simulink model "RVC_Joint_space_PD_control_gravity_compensation"  (R2020b)
settings: Solver=VariableStepAuto  StartTime=0.0  StopTime=5  RelTol=1e-3
values from neighbouring files (symbols this model uses):
  gravity = [0 0 9.81]'    [RVC_main.m]
  KD_J = diag([1 1 1 0.1 0.1 0.1])    [RVC_main.m]
  KP_J = diag([0.5 0.5 0.5 0.25 0.255 0.25])    [RVC_main.m]
undefined symbols (not defined in the file or in its folder): dh, inv_dyn_recursive_NewtonEulero
libraries: vrlib x1
settings Model: Creator=eros  LastModifiedBy=Edoardo

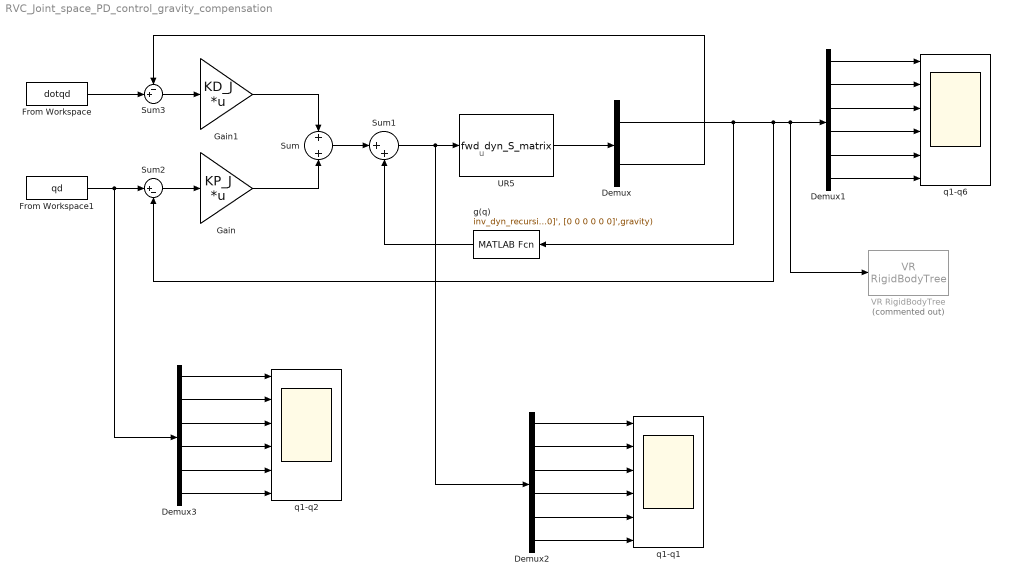
== system RVC_Joint_space_PD_control_gravity_compensation ==
  note: u
  Demux : Demux  Outputs=2
  Demux1 : Demux  Outputs=dh.dof
  Demux2 : Demux  Outputs=dh.dof
  Demux3 : Demux  Outputs=dh.dof
  From Workspace : FromWorkspace  VariableName=dotqd
  From Workspace1 : FromWorkspace  VariableName=qd
  Gain : Gain  Gain=KP_J  Multiplication=Matrix(K*u)
  Gain1 : Gain  Gain=KD_J  Multiplication=Matrix(K*u)
  Sum : Sum
  Sum1 : Sum  Inputs=|++
  Sum2 : Sum  Inputs=|+-
  Sum3 : Sum  Inputs=-+|
  UR5 : S-Function  FunctionName=fwd_dyn_S_matrix  Parameters=dh, he, gravity, q0, dotq0  SFunctionDeploymentMode=off  EnableBusSupport=off
  VR RigidBodyTree : vrlib/VR RigidBodyTree  Commented=on  RBT=UR5_robot  useRBT=on  Ts=-1  ForceViewerOpen=on
      settings: SourceProductBaseCode=SL
  g(q) : MATLABFcn  MATLABFcn=inv_dyn_recursive_NewtonEulero(dh,u,[0 0 0 0 0 0]', [0 0 0 0 0 0]',gravity)  OutputDimensions=[dh.dof 1]  Output1D=off
  q1-q1 : Scope  NumInputPorts=6
  q1-q2 : Scope  NumInputPorts=6
  q1-q6 : Scope  NumInputPorts=6
  wires:
  Sum/1 -> Sum1/1
  g(q)/1 -> Sum1/2
  Gain/1 -> Sum/2
  UR5/1 -> Demux/1
  Demux/1 -> Sum2/2, VR RigidBodyTree/1, Demux1/1, g(q)/1
  Sum2/1 -> Gain/1
  Gain1/1 -> Sum/1
  Demux1/1 -> q1-q6/1
  Demux1/2 -> q1-q6/2
  Demux1/3 -> q1-q6/3
  Demux1/4 -> q1-q6/4
  Demux1/5 -> q1-q6/5
  Demux1/6 -> q1-q6/6
  From Workspace/1 -> Sum3/2
  Demux/2 -> Sum3/1
  Sum3/1 -> Gain1/1
  Demux2/3 -> q1-q1/3
  Demux2/1 -> q1-q1/1
  Demux2/5 -> q1-q1/5
  Demux2/4 -> q1-q1/4
  Sum1/1 -> Demux2/1, UR5/1
  Demux2/6 -> q1-q1/6
  Demux2/2 -> q1-q1/2
  Demux3/2 -> q1-q2/2
  From Workspace1/1 -> Demux3/1, Sum2/1
  Demux3/4 -> q1-q2/4
  Demux3/1 -> q1-q2/1
  Demux3/5 -> q1-q2/5
  Demux3/6 -> q1-q2/6
  Demux3/3 -> q1-q2/3
